simulink subsystem "tehrani_tissue_compartment"  (R2019b)
settings: Solver=VariableStepAuto  StartTime=0.0  StopTime=10.0  RelTol=1e-3
undefined symbols (not defined in the file): __PRM__SERIALIZED__DATA__, C_v_CO2_0, C_v_O2_0, SubsystemReferenceBlock
settings Model: Creator=RH  LastModifiedBy=RH

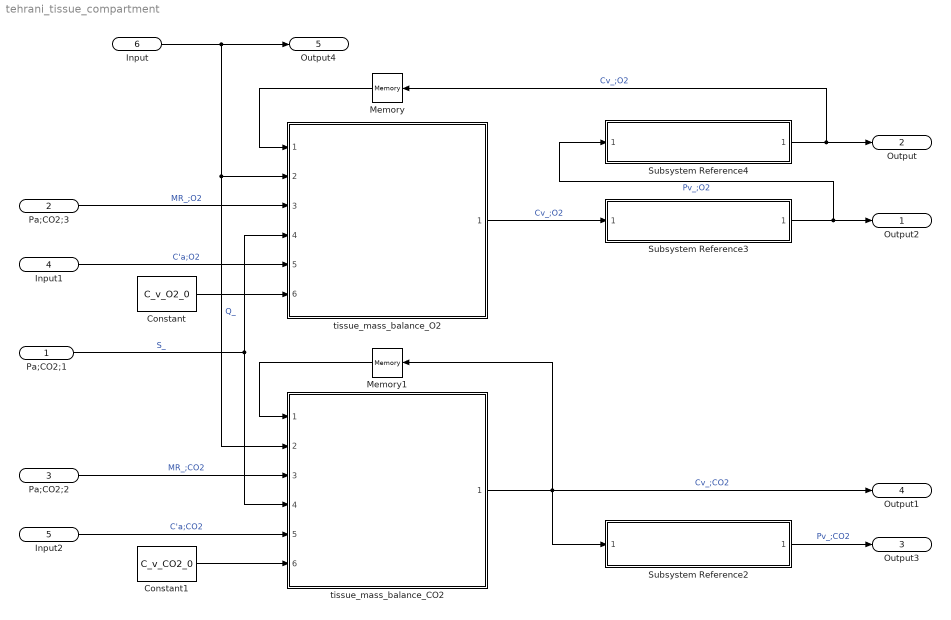
== system tehrani_tissue_compartment ==
  Pa;CO2;1 : Inport  Unit=liter
  Pa;CO2;3 : Inport  Port=2  Unit=liter/second
  Pa;CO2;2 : Inport  Port=3  Unit=liter/second
  Input1 : Inport  Port=4  Unit=1
  Input2 : Inport  Port=5  Unit=1
  Input : Inport  Port=6  Unit=L/min
  Constant : Constant  Value=C_v_O2_0
  Constant1 : Constant  Value=C_v_CO2_0
  Memory : Memory
  Memory1 : Memory
  Subsystem Reference2 : Subsystem  BlockKeywords=__PRM__SERIALIZED__DATA__:SubsystemReferenceBlock  ReferencedSubsystem=CO2_dissociation_inv
  Subsystem Reference3 : Subsystem  BlockKeywords=__PRM__SERIALIZED__DATA__:SubsystemReferenceBlock  ReferencedSubsystem=O2_dissociation_inv
  Subsystem Reference4 : Subsystem  BlockKeywords=__PRM__SERIALIZED__DATA__:SubsystemReferenceBlock  ReferencedSubsystem=O2_dissociation
  tissue_mass_balance_CO2 : Subsystem  ReferencedSubsystem=tehrani_tissue_mass_balance_v2
  tissue_mass_balance_O2 : Subsystem  ReferencedSubsystem=tehrani_tissue_mass_balance_v2
  Output2 : Outport  Unit=mmHg
  Output : Outport  Port=2  Unit=1
  Output3 : Outport  Port=3  Unit=mmHg
  Output1 : Outport  Port=4  Unit=1
  Output4 : Outport  Port=5  Unit=liter/minute
  wires:
  Subsystem Reference3/1 -> Output2/1, Subsystem Reference4/1  "Pv_;O2"
  Subsystem Reference2/1 -> Output3/1  "Pv_;CO2"
  Input/1 -> Output4/1, tissue_mass_balance_O2/2, tissue_mass_balance_CO2/2  "Q_"
  Pa;CO2;3/1 -> tissue_mass_balance_O2/3  "MR_;O2"
  Pa;CO2;2/1 -> tissue_mass_balance_CO2/3  "MR_;CO2"
  Pa;CO2;1/1 -> tissue_mass_balance_CO2/4, tissue_mass_balance_O2/4  "S_"
  tissue_mass_balance_CO2/1 -> Memory1/1, Output1/1, Subsystem Reference2/1  "Cv_;CO2"
  Input1/1 -> tissue_mass_balance_O2/5  "C'a;O2"
  Input2/1 -> tissue_mass_balance_CO2/5  "C'a;CO2"
  tissue_mass_balance_O2/1 -> Subsystem Reference3/1  "Cv_;O2"
  Constant/1 -> tissue_mass_balance_O2/6
  Constant1/1 -> tissue_mass_balance_CO2/6
  Memory/1 -> tissue_mass_balance_O2/1
  Subsystem Reference4/1 -> Output/1, Memory/1  "Cv_;O2"
  Memory1/1 -> tissue_mass_balance_CO2/1
